simulink model "dis_try_1"  (Simulink 8.7)
settings: Solver=FixedStepAuto  StartTime=0.0  StopTime=10.0  RelTol=1e-3
settings Model: Creator=Godric  LastModifiedBy=Godric
settings DataIOCC: LimitDataPoints=off  SaveFormat=Dataset
settings DebuggingCC: UnderspecifiedInitializationDetection=Simplified  MergeDetectMultiDrivingBlocksExec=error
settings HardwareCC: ProdBitPerPointer=64  ProdLargestAtomicFloat=Float  ProdIntDivRoundTo=Zero  ProdEndianess=LittleEndian  ProdWordSize=64  ProdHWDeviceType=Intel->x86-64 (Windows64)
settings ModelReferenceCC: PropagateSignalLabelsOutOfModel=on
settings ConfigComp: CovModelRefEnable=off

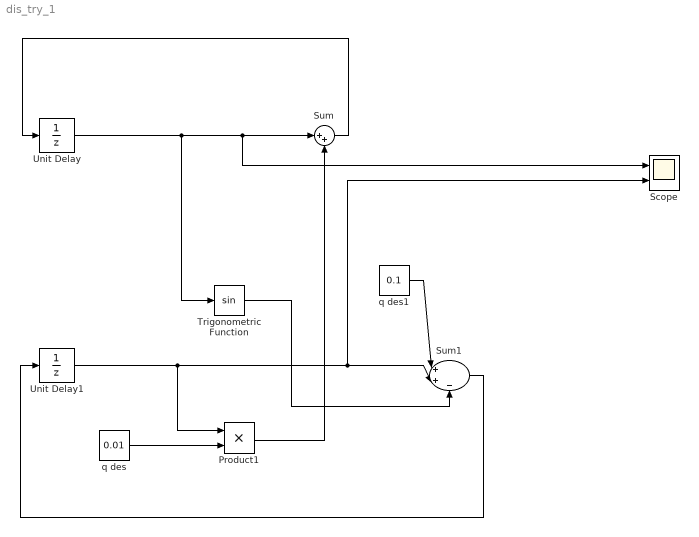
== system dis_try_1 ==
  Product1 : Product
  Scope : Scope  NumInputPorts=2
  Sum : Sum  Inputs=|++
  Sum1 : Sum  Inputs=|++-
  Trigonometric Function : Trigonometry
  Unit Delay : UnitDelay  InitialCondition=0.5  SampleTime=-1
  Unit Delay1 : UnitDelay  InitialCondition=0.5  SampleTime=-1
  q des : Constant  Value=0.01
  q des1 : Constant  Value=0.1
  wires:
  Sum/1 -> Unit Delay/1
  Unit Delay/1 -> Trigonometric Function/1, Scope/1, Sum/1
  q des/1 -> Product1/2
  Unit Delay1/1 -> Scope/2, Sum1/2, Product1/1
  Product1/1 -> Sum/2
  Trigonometric Function/1 -> Sum1/3
  q des1/1 -> Sum1/1
  Sum1/1 -> Unit Delay1/1
